simulink model "plant_block_Conrad"  (R2019b)
settings: Solver=ode1  StartTime=0.0  StopTime=700  RelTol=1e-3  EnableMultiTasking=on
undefined symbols (not defined in the file or in its folder): K4
libraries: simulink x8
settings Model: SimulationMode=external  Creator=Dro  LastModifiedBy=s4479115
settings DataIOCC: LimitDataPoints=on  SaveFormat=Array  ReturnWorkspaceOutputs=off  SignalLoggingName=sigsOut
settings OptimizationCC: ExpressionDepthLimit=2147483647  InitFltsAndDblsToZero=on
settings DebuggingCC: SaveWithParameterizedLinksMsg=none  UnderspecifiedInitializationDetection=Classic  MergeDetectMultiDrivingBlocksExec=none  SignalResolutionControl=TryResolveAllWithWarning  MultiTaskDSMMsg=warning  MultiTaskCondExecSysMsg=none  FcnCallInpInsideContextMsg=warning  StateNameClashWarn=warning  SFUnexpectedBacktrackingDiag=warning  SFNoUnconditionalDefaultTransitionDiag=warning  SFExecutionAtInitializationDiag=none  ArithmeticOperatorsInVariantConditions=warning
settings HardwareCC: TargetBitPerLong=64  TargetBitPerPointer=64  TargetIntDivRoundTo=Zero  TargetEndianess=LittleEndian  TargetWordSize=64  TargetHWDeviceType=Intel->x86-64
settings ModelReferenceCC: PropagateSignalLabelsOutOfModel=off
settings SFSimCC: SimUseLocalCustomCode=off  CustomCodeUndefinedFunction=UseInterfaceOnly
settings RTWCC: Description=Simulink Desktop Real-Time  SystemTargetFile=sldrt.tlc  TemplateMakefile=sldrt.tmf  RTWUseLocalCustomCode=off  RTWCompilerOptimization=on
settings CodeAppCC: MaxIdLength=95  StateflowObjectComments=on
settings SimulinkDesktopRealTimeCC: TargetPreCompLibLocation=C:\Program Files\MATLAB\R2019b\toolbox\sldrt\lib\win64  TargetLangStandard=C89/C90 (ANSI)  ModelReferenceCompliant=off  CompOptLevelCompliant=off  SupportVariableSizeSignals=off  PreserveStateflowLocalDataDimensions=off
settings ConfigComp: CovMetricSettings=dw  CovHtmlReporting=on  CovSaveCumulativeToWorkspaceVar=on  CovSaveSingleToWorkspaceVar=on  CovExternalEMLEnable=off

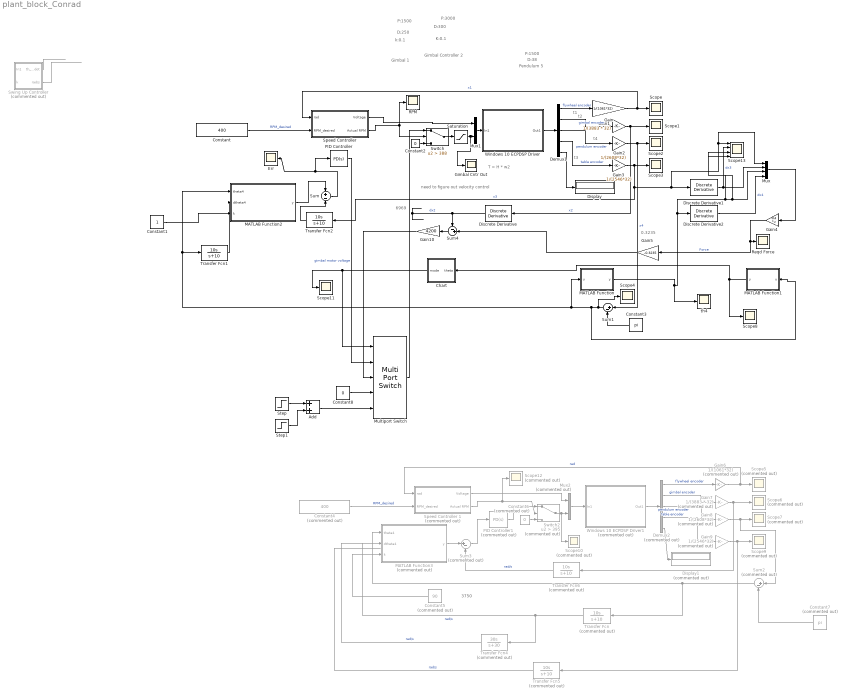
== system plant_block_Conrad ==
  note: 6969
  note: need to figure out velocity control
  note: 3750
  note: Pendulum 5
  note: D:38
  note: P:1500
  note: 0.3235
  note: t3
  note: t4
  note: t2
  note: t1
  note: T = H * w2
  note: Gimbal Controller 2
  note: K:0.1
  note: D:300
  note: P:3000
  note: Gimbal 1
  note: k:0.1
  note: D:250
  note: P:1500
  Add : Sum
  Chart : Stateflow chart  BlockKeywords=__PRM__SERIALIZED__DATA__:Stateflow Chart,Stateflow Diagram  TreatAsAtomicUnit=on
  Constant : Constant  Value=400
  Constant1 : Constant
  Constant2 : Constant  Value=0
  Constant3 : Constant  Value=pi
  Constant4 : Constant  Commented=on  Value=400
  Constant5 : Constant  Commented=on  Value=90  VectorParams1D=off
  Constant6 : Constant  Commented=on  Value=0
  Constant7 : Constant  Commented=on  Value=pi
  Constant8 : Constant  Value=0
  Demux1 : Demux  Outputs=5
  Demux2 : Demux  Commented=on  Outputs=5
  Discrete Derivative : simulink/Discrete/Discrete Derivative  gainval=1.0  ICPrevScaledInput=0.0  OutMin=[]  OutMax=[]  OutDataType=fixdt(1, 16)  OutScaling=2^-10  DoSatur=off
  Discrete Derivative1 : simulink/Discrete/Discrete Derivative  gainval=1.0  ICPrevScaledInput=0.0  OutMin=[]  OutMax=[]  OutDataType=fixdt(1, 16)  OutScaling=2^-10  DoSatur=off
  Discrete Derivative2 : simulink/Discrete/Discrete Derivative  gainval=1.0  ICPrevScaledInput=0.0  OutMin=[]  OutMax=[]  OutDataType=fixdt(1, 16)  OutScaling=2^-10  DoSatur=off
  Display : Display
  Display1 : Display  Commented=on
  Err : Scope
  Gain : Gain  Gain=1/(1061*32)
  Gain1 : Gain  Gain=1/(3883 * 32)
  Gain10 : Gain  Gain=4200
  Gain2 : Gain  Gain=1/(2608*32)
  Gain3 : Gain  Gain=1/(2546*32)
  Gain4 : Gain  Gain=-K4  Multiplication=Matrix(K*u)
  Gain5 : Gain  Gain=-0.3235
  Gain6 : Gain  Commented=on  Gain=1/(1061*32)
  Gain7 : Gain  Commented=on  Gain=1/(3883 * 32)
  Gain8 : Gain  Commented=on  Gain=1/(2608*32)
  Gain9 : Gain  Commented=on  Gain=1/(2546*32)
  Gimbal Cntr Out : Scope
  MATLAB Function : MATLAB Function  TreatAsAtomicUnit=on
  MATLAB Function1 : MATLAB Function  TreatAsAtomicUnit=on
  MATLAB Function2 : MATLAB Function  TreatAsAtomicUnit=on
  MATLAB Function3 : MATLAB Function  Commented=on  TreatAsAtomicUnit=on
  Multiport Switch : MultiPortSwitch  Inputs=4
  Mux : Mux
  Mux1 : Mux  Inputs=2
  Mux2 : Mux  Commented=on  Inputs=2
  PID Controller : simulink/Continuous/PID Controller  Controller=PD  Form=Parallel  TimeDomain=Continuous-time  SampleTime=-1  IntegratorMethod=Forward Euler  FilterMethod=Forward Euler  ControllerParametersSource=internal  P=4000  I=0  D=0  UseFilter=on  N=100  TunerSelectOption=Transfer Function Based (PID Tuner App)  InitialConditionSource=internal  InitialConditionForIntegrator=0  InitialConditionForFilter=0  DifferentiatorICPrevScaledInput=0  ExternalReset=none  TrackingMode=off  Kt=1  LimitOutput=off  UpperSaturationLimit=inf  LowerSaturationLimit=-inf  LinearizeAsGain=on  AntiWindupMode=none  Kb=1  POutMin=[]  POutMax=[]  IOutMin=[]  IOutMax=[]  DOutMin=[]  DOutMax=[]  NOutMin=[]  NOutMax=[]  SumOutMin=[]  SumOutMax=[]  SaturationOutMin=[]  SaturationOutMax=[]  PParamMin=[]  PParamMax=[]  IParamMin=[]  IParamMax=[]  DParamMin=[]  DParamMax=[]  NParamMin=[]  NParamMax=[]  KbParamMin=[]  KbParamMax=[]  KtParamMin=[]  KtParamMax=[]  KbOutMin=[]  KbOutMax=[]  KtOutMin=[]  KtOutMax=[]  IntegratorOutMin=[]  IntegratorOutMax=[]  FilterOutMin=[]  FilterOutMax=[]  SumI1OutMin=[]  SumI1OutMax=[]  SumI2OutMin=[]  SumI2OutMax=[]  SumI3OutMin=[]  SumI3OutMax=[]  SumI4OutMin=[]  SumI4OutMax=[]  SumDOutMin=[]  SumDOutMax=[]  DifferentiatorOutMin=[]  DifferentiatorOutMax=[]  FilterDiffOutCoefMin=[]  FilterDiffOutCoefMax=[]  ReciprocalOutMin=[]  ReciprocalOutMax=[]  SumDenOutMin=[]  SumDenOutMax=[]  SumNumOutMin=[]  SumNumOutMax=[]  DivideOutMin=[]  DivideOutMax=[]  IntegratorContinuousStateAttributes=''  IntegratorStateMustResolveToSignalObject=off  IntegratorRTWStateStorageClass=Auto  FilterContinuousStateAttributes=''  FilterStateMustResolveToSignalObject=off  FilterRTWStateStorageClass=Auto  ParallelPVariant=InternalParameters  IdealPVariant=Disabled  IVariant=Disabled  DVariant=InternalParameters  IntegratorVariant=Disabled  SatVariant=Disabled  AWVariant=Disabled  PCopyVariant=Disabled  TRVariant=Disabled  FdbkBlocksVariant=Forward  IdealPFdbkVariant=Disabled  SatFdbkVariant=Disabled  DerivativeFilterVariant=ContFilter  NVariant=InternalParameters  NCopyVariant=Disabled  FilterICVariant=InternalICsFilter  IntegratorICVariant=Disabled  ExternalResetVariant=Disabled  TRSumVariant=Passthrough  SumFdbkVariant=Disabled  SumVariant=Sum_PD
  PID Controller1 : simulink/Continuous/PID Controller  Commented=on  Controller=PD  Form=Parallel  TimeDomain=Continuous-time  SampleTime=-1  IntegratorMethod=Forward Euler  FilterMethod=Forward Euler  ControllerParametersSource=internal  P=40  I=1  D=0.05  UseFilter=on  N=100  TunerSelectOption=Transfer Function Based (PID Tuner App)  InitialConditionSource=internal  InitialConditionForIntegrator=0  InitialConditionForFilter=0  DifferentiatorICPrevScaledInput=0  ExternalReset=none  TrackingMode=off  Kt=1  LimitOutput=off  UpperSaturationLimit=inf  LowerSaturationLimit=-inf  LinearizeAsGain=on  AntiWindupMode=none  Kb=1  POutMin=[]  POutMax=[]  IOutMin=[]  IOutMax=[]  DOutMin=[]  DOutMax=[]  NOutMin=[]  NOutMax=[]  SumOutMin=[]  SumOutMax=[]  SaturationOutMin=[]  SaturationOutMax=[]  PParamMin=[]  PParamMax=[]  IParamMin=[]  IParamMax=[]  DParamMin=[]  DParamMax=[]  NParamMin=[]  NParamMax=[]  KbParamMin=[]  KbParamMax=[]  KtParamMin=[]  KtParamMax=[]  KbOutMin=[]  KbOutMax=[]  KtOutMin=[]  KtOutMax=[]  IntegratorOutMin=[]  IntegratorOutMax=[]  FilterOutMin=[]  FilterOutMax=[]  SumI1OutMin=[]  SumI1OutMax=[]  SumI2OutMin=[]  SumI2OutMax=[]  SumI3OutMin=[]  SumI3OutMax=[]  SumI4OutMin=[]  SumI4OutMax=[]  SumDOutMin=[]  SumDOutMax=[]  DifferentiatorOutMin=[]  DifferentiatorOutMax=[]  FilterDiffOutCoefMin=[]  FilterDiffOutCoefMax=[]  ReciprocalOutMin=[]  ReciprocalOutMax=[]  SumDenOutMin=[]  SumDenOutMax=[]  SumNumOutMin=[]  SumNumOutMax=[]  DivideOutMin=[]  DivideOutMax=[]  IntegratorContinuousStateAttributes=''  IntegratorStateMustResolveToSignalObject=off  IntegratorRTWStateStorageClass=Auto  FilterContinuousStateAttributes=''  FilterStateMustResolveToSignalObject=off  FilterRTWStateStorageClass=Auto  ParallelPVariant=InternalParameters  IdealPVariant=Disabled  IVariant=Disabled  DVariant=InternalParameters  IntegratorVariant=Disabled  SatVariant=Disabled  AWVariant=Disabled  PCopyVariant=Disabled  TRVariant=Disabled  FdbkBlocksVariant=Forward  IdealPFdbkVariant=Disabled  SatFdbkVariant=Disabled  DerivativeFilterVariant=ContFilter  NVariant=InternalParameters  NCopyVariant=Disabled  FilterICVariant=InternalICsFilter  IntegratorICVariant=Disabled  ExternalResetVariant=Disabled  TRSumVariant=Passthrough  SumFdbkVariant=Disabled  SumVariant=Sum_PD
  "RPM " : Scope
  Reqd Force : Scope
  Saturation : Saturate  UpperLimit=16000  LowerLimit=-16000
  Scope{,1..4,8,11} (7 alike) : Scope
  Scope{5..7,9..10,12} (6 alike) : Scope  Commented=on
  Scope13 : Scope  NumInputPorts=4
  "Speed Controller " : Subsystem
  Speed Controller 1 : Subsystem  Commented=on
  Step : Step  Time=30  After=3000  SampleTime=0
  Step1 : Step  Time=30.2  Before=3000  After=-3000  SampleTime=0
  Sum : Sum  Inputs=+-
  Sum1 : Sum  Inputs=|+-
  Sum2 : Sum  Commented=on  Inputs=|+-
  Sum3 : Sum  Commented=on  Inputs=|+-
  Sum4 : Sum  Inputs=-+|
  "Swing Up Controller " : Subsystem  Commented=on
  Switch : Switch  Criteria=u2 > Threshold  Threshold=388
  Switch2 : Switch  Commented=on  Criteria=u2 > Threshold  Threshold=395
  Transfer Fcn : TransferFcn  Commented=on  Numerator=[10 0 ]  Denominator=[1 10]
  Transfer Fcn1 : TransferFcn  Numerator=[10 0]  Denominator=[1 10]
  Transfer Fcn2 : TransferFcn  Numerator=[10 0]  Denominator=[1 10]
  Transfer Fcn4 : TransferFcn  Commented=on  Numerator=[30 0 ]  Denominator=[1 30]
  Transfer Fcn5 : TransferFcn  Commented=on  Numerator=[10 0 ]  Denominator=[1 10]
  Transfer Fcn6 : TransferFcn  Commented=on  Numerator=[10 0 ]  Denominator=[1 10]
  Windows 10 ECPDSP Driver : Subsystem  mask{BaseAddr='0x3F00', STime=0.008, TimeOutPer=500, HWAccess=on}
      mask prompts: BaseAddr "Base I/O Address"; STime "Sample Time (Sec)"; TimeOutPer "Timeout Period (500 ~ 2000)"; HWAccess "Hardware Access"
      mask Display: color('black');disp('ECPDSP Driver\n upto\n 4 Encs(ADC Channels)\n and 2 Dacs')
  Windows 10 ECPDSP Driver1 : Subsystem  Commented=on  mask{BaseAddr='0x3F00', STime=0.008, TimeOutPer=500, HWAccess=on}
      mask prompts: BaseAddr "Base I/O Address"; STime "Sample Time (Sec)"; TimeOutPer "Timeout Period (500 ~ 2000)"; HWAccess "Hardware Access"
      mask Display: color('black');disp('ECPDSP Driver\n upto\n 4 Encs(ADC Channels)\n and 2 Dacs')
  th4 : Scope
  wires:
  Mux1/1 -> Windows 10 ECPDSP Driver/1(In1)
  Demux1/1 -> Gain/1  "flywheel encoder"
  Demux1/2 -> Gain1/1  "gimbal encoder"
  Demux1/3 -> Gain2/1  "pendulum encoder"
  Demux1/4 -> Gain3/1  "table encoder"
  Gain4/1 -> Gain5/1, Reqd Force/1  "Force"
  Windows 10 ECPDSP Driver/1(Out1) -> Demux1/1
  Demux1/5 -> Display/1
  Gain/1 -> "Speed Controller "/1(rad), Scope/1  "x1"
  Gain1/1 -> Discrete Derivative/1, Scope1/1  "x2"
  Gain3/1 -> Transfer Fcn2/1, Discrete Derivative1/1, Scope13/1, Mux/1, Scope3/1  "x3"
  Constant/1 -> "Speed Controller "/2(RPM_desired)  "RPM_desired"
  "Speed Controller "/1(Voltage) -> Mux1/1
  "Speed Controller "/2("Actual RPM ") -> "RPM "/1, Switch/2
  Constant2/1 -> Switch/3
  Constant3/1 -> Sum1/2
  Gain2/1 -> Sum1/1, Scope2/1  "x4"
  Discrete Derivative2/1 -> Mux/4  "dx4"
  Discrete Derivative1/1 -> Scope13/2, Mux/2  "dx3"
  Mux/1 -> Gain4/1
  MATLAB Function1/1(y) -> Chart/1(theta), Scope8/1
  PID Controller/1 -> Multiport Switch/2  "gimbal motor voltage"
  Discrete Derivative/1 -> Sum4/1  "dx2"
  Gain5/1 -> Sum4/2
  "Swing Up Controller "/1(th_2_dot) -> ?
  Constant1/1 -> MATLAB Function2/3(k)
  "Swing Up Controller "/2(rad/s) -> ?
  Chart/1(mode) -> Multiport Switch/1, Scope11/1
  Sum/1 -> Err/1, PID Controller/1
  Sum1/1 -> Scope4/1, MATLAB Function2/1(theta4), Transfer Fcn1/1, MATLAB Function/1(u), MATLAB Function1/1(u)
  MATLAB Function/1(y) -> th4/1, Discrete Derivative2/1, Scope13/3, Scope13/4, Mux/3
  Speed Controller 1/1(Voltage) -> Mux2/1
  Transfer Fcn5/1 -> ?  "rad/s"
  Gain9/1 -> Transfer Fcn5/1, Scope9/1
  Transfer Fcn4/1 -> ?  "rad/s"
  Transfer Fcn/1 -> MATLAB Function3/2(dtheta4), Transfer Fcn4/1  "rad/s"
  Mux2/1 -> Windows 10 ECPDSP Driver1/1(In1)
  Demux2/3 -> Gain8/1  "pendulum encoder"
  Windows 10 ECPDSP Driver1/1(Out1) -> Demux2/1
  Constant4/1 -> Speed Controller 1/2(RPM_desired)  "RPM_desired"
  Gain6/1 -> Speed Controller 1/1(rad), Scope5/1  "rad"
  Sum2/1 -> MATLAB Function3/1(theta4), Transfer Fcn/1
  Switch2/1 -> Scope10/1, Mux2/2
  Speed Controller 1/2("Actual RPM ") -> Scope12/1, Switch2/2
  Demux2/2 -> Gain7/1  "gimbal encoder"
  Demux2/4 -> Gain9/1  "table encoder"
  Demux2/5 -> Display1/1
  Gain7/1 -> Transfer Fcn6/1, Scope6/1
  Constant6/1 -> Switch2/3
  Constant5/1 -> MATLAB Function3/3(k)
  Gain8/1 -> Scope7/1, Sum2/1
  Constant7/1 -> Sum2/2
  Demux2/1 -> Gain6/1  "flywheel encoder"
  MATLAB Function3/1(y) -> Sum3/1
  PID Controller1/1 -> Switch2/1
  Sum3/1 -> PID Controller1/1
  Transfer Fcn6/1 -> Sum3/2  "rad/s"
  Gain10/1 -> Multiport Switch/3
  Multiport Switch/1 -> Switch/1
  Switch/1 -> Saturation/1
  Saturation/1 -> Gimbal Cntr Out/1, Mux1/2
  Sum4/1 -> Gain10/1
  MATLAB Function2/1(y) -> Sum/1
  Transfer Fcn1/1 -> MATLAB Function2/2(dtheta4)
  Transfer Fcn2/1 -> Sum/2
  Constant8/1 -> Multiport Switch/4
  Add/1 -> Multiport Switch/5
  Step/1 -> Add/1
  Step1/1 -> Add/2

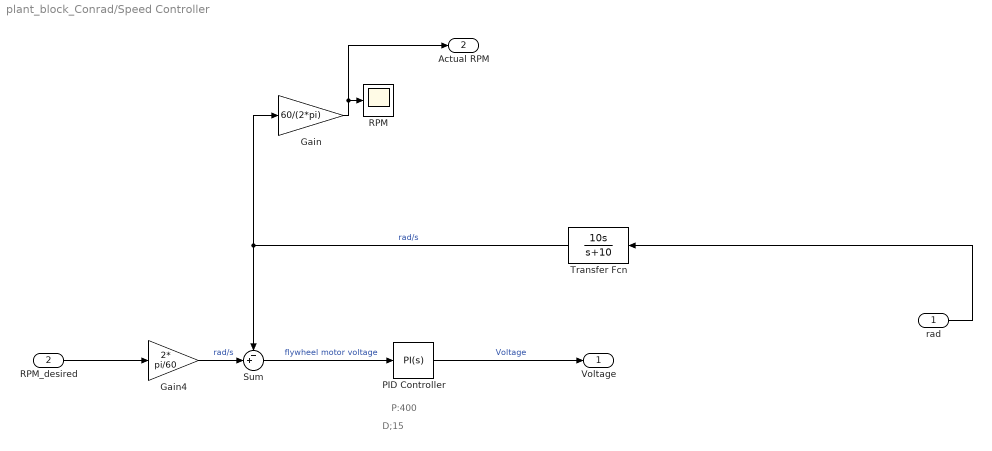
== system plant_block_Conrad/Speed Controller  ==
  note: D;15
  note: P:400
  rad : Inport
  RPM_desired : Inport  Port=2
  Gain : Gain  Gain=60/(2*pi)
  Gain4 : Gain  Gain=2* pi/60
  PID Controller : simulink/Continuous/PID Controller  Controller=PI  Form=Parallel  TimeDomain=Continuous-time  SampleTime=-1  IntegratorMethod=Forward Euler  FilterMethod=Forward Euler  ControllerParametersSource=internal  P=390  I=15  D=0  UseFilter=on  N=100  TunerSelectOption=Transfer Function Based (PID Tuner App)  InitialConditionSource=internal  InitialConditionForIntegrator=0  InitialConditionForFilter=0  DifferentiatorICPrevScaledInput=0  ExternalReset=none  TrackingMode=off  Kt=1  LimitOutput=off  UpperSaturationLimit=inf  LowerSaturationLimit=-inf  LinearizeAsGain=on  AntiWindupMode=none  Kb=1  POutMin=[]  POutMax=[]  IOutMin=[]  IOutMax=[]  DOutMin=[]  DOutMax=[]  NOutMin=[]  NOutMax=[]  SumOutMin=[]  SumOutMax=[]  SaturationOutMin=[]  SaturationOutMax=[]  PParamMin=[]  PParamMax=[]  IParamMin=[]  IParamMax=[]  DParamMin=[]  DParamMax=[]  NParamMin=[]  NParamMax=[]  KbParamMin=[]  KbParamMax=[]  KtParamMin=[]  KtParamMax=[]  KbOutMin=[]  KbOutMax=[]  KtOutMin=[]  KtOutMax=[]  IntegratorOutMin=[]  IntegratorOutMax=[]  FilterOutMin=[]  FilterOutMax=[]  SumI1OutMin=[]  SumI1OutMax=[]  SumI2OutMin=[]  SumI2OutMax=[]  SumI3OutMin=[]  SumI3OutMax=[]  SumI4OutMin=[]  SumI4OutMax=[]  SumDOutMin=[]  SumDOutMax=[]  DifferentiatorOutMin=[]  DifferentiatorOutMax=[]  FilterDiffOutCoefMin=[]  FilterDiffOutCoefMax=[]  ReciprocalOutMin=[]  ReciprocalOutMax=[]  SumDenOutMin=[]  SumDenOutMax=[]  SumNumOutMin=[]  SumNumOutMax=[]  DivideOutMin=[]  DivideOutMax=[]  IntegratorContinuousStateAttributes=''  IntegratorStateMustResolveToSignalObject=off  IntegratorRTWStateStorageClass=Auto  FilterContinuousStateAttributes=''  FilterStateMustResolveToSignalObject=off  FilterRTWStateStorageClass=Auto  ParallelPVariant=InternalParameters  IdealPVariant=Disabled  IVariant=InternalParameters  DVariant=Disabled  IntegratorVariant=Continuous  SatVariant=Disabled  AWVariant=Passthrough  PCopyVariant=Disabled  TRVariant=Disabled  FdbkBlocksVariant=Forward  IdealPFdbkVariant=Disabled  SatFdbkVariant=Disabled  DerivativeFilterVariant=Disabled  NVariant=Disabled  NCopyVariant=Disabled_SignalSpec  FilterICVariant=Disabled  IntegratorICVariant=InternalICs  ExternalResetVariant=Disabled  TRSumVariant=Passthrough  SumFdbkVariant=Disabled  SumVariant=Sum_PI
  RPM : Scope
  Sum : Sum  Inputs=-+|
  Transfer Fcn : TransferFcn  Numerator=[10 0 ]  Denominator=[1 10]
  Voltage : Outport
  "Actual RPM " : Outport  Port=2
  wires:
  Gain4/1 -> Sum/2  "rad/s"
  Transfer Fcn/1 -> Gain/1, Sum/1  "rad/s"
  Sum/1 -> PID Controller/1  "flywheel motor voltage"
  PID Controller/1 -> Voltage/1  "Voltage"
  RPM_desired/1 -> Gain4/1
  rad/1 -> Transfer Fcn/1
  Gain/1 -> "Actual RPM "/1, RPM/1

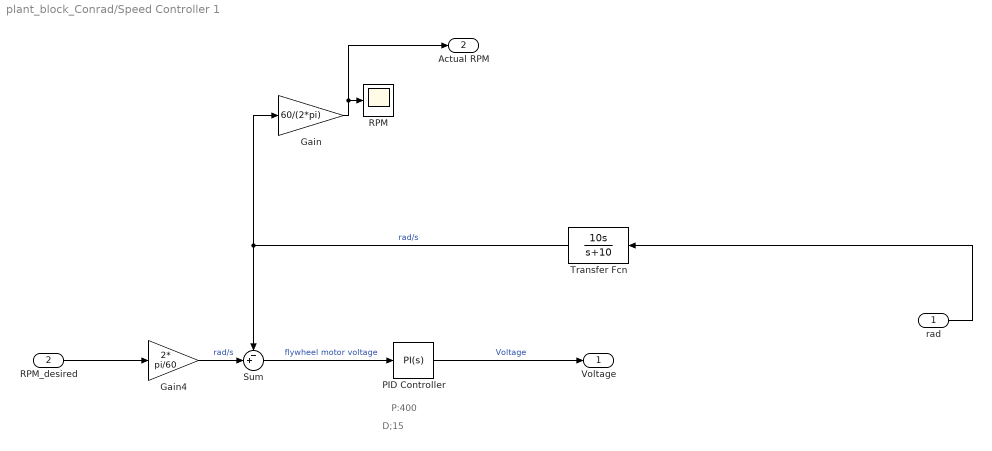
== system plant_block_Conrad/Speed Controller 1 ==
  note: D;15
  note: P:400
  rad : Inport
  RPM_desired : Inport  Port=2
  Gain : Gain  Gain=60/(2*pi)
  Gain4 : Gain  Gain=2* pi/60
  PID Controller : simulink/Continuous/PID Controller  Controller=PI  Form=Parallel  TimeDomain=Continuous-time  SampleTime=-1  IntegratorMethod=Forward Euler  FilterMethod=Forward Euler  ControllerParametersSource=internal  P=600  I=50  D=0  UseFilter=on  N=100  TunerSelectOption=Transfer Function Based (PID Tuner App)  InitialConditionSource=internal  InitialConditionForIntegrator=0  InitialConditionForFilter=0  DifferentiatorICPrevScaledInput=0  ExternalReset=none  TrackingMode=off  Kt=1  LimitOutput=off  UpperSaturationLimit=inf  LowerSaturationLimit=-inf  LinearizeAsGain=on  AntiWindupMode=none  Kb=1  POutMin=[]  POutMax=[]  IOutMin=[]  IOutMax=[]  DOutMin=[]  DOutMax=[]  NOutMin=[]  NOutMax=[]  SumOutMin=[]  SumOutMax=[]  SaturationOutMin=[]  SaturationOutMax=[]  PParamMin=[]  PParamMax=[]  IParamMin=[]  IParamMax=[]  DParamMin=[]  DParamMax=[]  NParamMin=[]  NParamMax=[]  KbParamMin=[]  KbParamMax=[]  KtParamMin=[]  KtParamMax=[]  KbOutMin=[]  KbOutMax=[]  KtOutMin=[]  KtOutMax=[]  IntegratorOutMin=[]  IntegratorOutMax=[]  FilterOutMin=[]  FilterOutMax=[]  SumI1OutMin=[]  SumI1OutMax=[]  SumI2OutMin=[]  SumI2OutMax=[]  SumI3OutMin=[]  SumI3OutMax=[]  SumI4OutMin=[]  SumI4OutMax=[]  SumDOutMin=[]  SumDOutMax=[]  DifferentiatorOutMin=[]  DifferentiatorOutMax=[]  FilterDiffOutCoefMin=[]  FilterDiffOutCoefMax=[]  ReciprocalOutMin=[]  ReciprocalOutMax=[]  SumDenOutMin=[]  SumDenOutMax=[]  SumNumOutMin=[]  SumNumOutMax=[]  DivideOutMin=[]  DivideOutMax=[]  IntegratorContinuousStateAttributes=''  IntegratorStateMustResolveToSignalObject=off  IntegratorRTWStateStorageClass=Auto  FilterContinuousStateAttributes=''  FilterStateMustResolveToSignalObject=off  FilterRTWStateStorageClass=Auto  ParallelPVariant=InternalParameters  IdealPVariant=Disabled  IVariant=InternalParameters  DVariant=Disabled  IntegratorVariant=Continuous  SatVariant=Disabled  AWVariant=Passthrough  PCopyVariant=Disabled  TRVariant=Disabled  FdbkBlocksVariant=Forward  IdealPFdbkVariant=Disabled  SatFdbkVariant=Disabled  DerivativeFilterVariant=Disabled  NVariant=Disabled  NCopyVariant=Disabled_SignalSpec  FilterICVariant=Disabled  IntegratorICVariant=InternalICs  ExternalResetVariant=Disabled  TRSumVariant=Passthrough  SumFdbkVariant=Disabled  SumVariant=Sum_PI
  RPM : Scope
  Sum : Sum  Inputs=-+|
  Transfer Fcn : TransferFcn  Numerator=[10 0 ]  Denominator=[1 10]
  Voltage : Outport
  "Actual RPM " : Outport  Port=2
  wires:
  Gain4/1 -> Sum/2  "rad/s"
  Transfer Fcn/1 -> Gain/1, Sum/1  "rad/s"
  Sum/1 -> PID Controller/1  "flywheel motor voltage"
  PID Controller/1 -> Voltage/1  "Voltage"
  RPM_desired/1 -> Gain4/1
  rad/1 -> Transfer Fcn/1
  Gain/1 -> "Actual RPM "/1, RPM/1

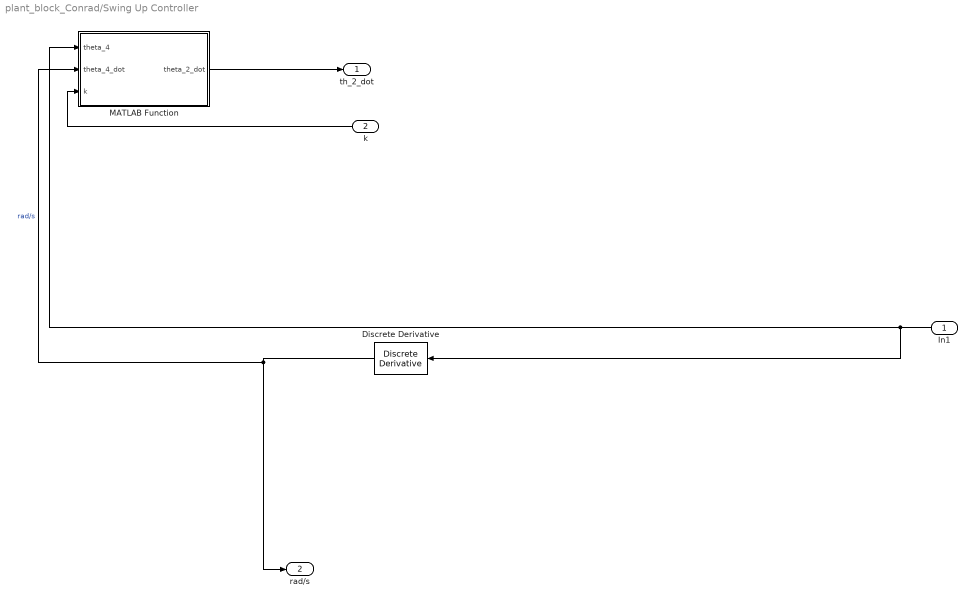
== system plant_block_Conrad/Swing Up Controller  ==
  In1 : Inport
  k : Inport  Port=2
  Discrete Derivative : simulink/Discrete/Discrete Derivative  gainval=1.0  ICPrevScaledInput=0.0  OutMin=[]  OutMax=[]  OutDataType=fixdt(1, 16)  OutScaling=2^-10  DoSatur=off
  MATLAB Function : MATLAB Function  TreatAsAtomicUnit=on
  th_2_dot : Outport
  rad/s : Outport  Port=2
  wires:
  MATLAB Function/1(theta_2_dot) -> th_2_dot/1
  k/1 -> MATLAB Function/3(k)
  Discrete Derivative/1 -> rad/s/1, MATLAB Function/2(theta_4_dot)  "rad/s"
  In1/1 -> Discrete Derivative/1, MATLAB Function/1(theta_4)

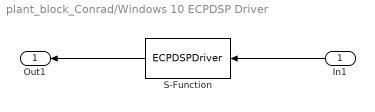
== system plant_block_Conrad/Windows 10 ECPDSP Driver ==
  In1 : Inport
  S-Function : S-Function  FunctionName=ECPDSPDriver  Parameters=BaseAddr,STime,TimeOutPer,HWAccess  SFunctionDeploymentMode=off  EnableBusSupport=off
  Out1 : Outport
  wires:
  In1/1 -> S-Function/1
  S-Function/1 -> Out1/1

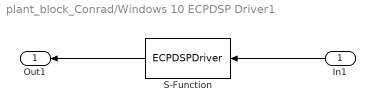
== system plant_block_Conrad/Windows 10 ECPDSP Driver1 ==
  In1 : Inport
  S-Function : S-Function  FunctionName=ECPDSPDriver  Parameters=BaseAddr,STime,TimeOutPer,HWAccess  SFunctionDeploymentMode=off  EnableBusSupport=off
  Out1 : Outport
  wires:
  In1/1 -> S-Function/1
  S-Function/1 -> Out1/1

== matlab function plant_block_Conrad/MATLAB Function1 ==
  data: u input; y output
function y = fcn(u)

y = min( abs(mod(u, 2 * pi)) , abs(mod(u, 2* pi) - 2 * pi));

== matlab function plant_block_Conrad/Swing Up Controller /MATLAB Function ==
  data: theta_4 input; theta_2_dot output; theta_4_dot input; k input
function theta_2_dot = fcn(theta_4, theta_4_dot, k)

theta_2_dot = -(36353776222982492160*k*theta_4_dot*cos(theta_4)*((3314449799178915*theta_4_dot^2)/576460752303423488 + (7532743254738029*cos(theta_4))/18014398509481984 - 7532743254738029/18014398509481984))/(299580375726665093*pi);
% theta_2_dot = -0.5722*k*theta_4_dot*cos(theta_4)*(0.0057*theta_4_dot^2 + 0.4182*cos(theta_4) - 0.4182);
end

== stateflow chart plant_block_Conrad/Chart ==
  state Spool1
    mode=3
  state Kick
    mode=4
  state Swing_up
    mode=1
  state Capture
    mode=2
  state Reset
    mode=3
  (default) -> Spool1
  Spool1 -> Kick : after(30000, msec)
  Swing_up -> Capture : [abs(theta)<0.08]
  Capture -> Reset : [abs(theta)>0.15]
  Kick -> Swing_up : after(500, msec)
  Reset -> Swing_up : after(3000, msec)
  data: mode output; theta input

== matlab function plant_block_Conrad/MATLAB Function ==
  data: u input; y output
function y = mabs(u)
% th = abs(u);
th1 = mod(u, 2 * pi);
th2 = 2*pi - th1;
arr = [th1, -th2];
[minMag, index] = min(abs(arr(:)));
y = minMag * sign(arr(index));
end

== matlab function plant_block_Conrad/MATLAB Function2 ==
  data: theta4 input; y output; dtheta4 input; k input
function y = fcn(theta4, dtheta4,k)
m = 0.1580;
lcg = 0.2698;
rh = 0.37;
J1 = 0.1314;
Jz_bar = 0.0131;
g = 9.81;
c = 0.002;
Eo = 0;
Id = 0.0148;
dtheta1 = 400 * (2*pi/60);

E = 0.5*m*lcg^2*dtheta4^2 + m*g*lcg*(cos(theta4) - 1);

% might need to negate k...simulation says so...???
y = -k*(E - Eo)*dtheta4*cos(theta4);

% dtheta2 = (rh/(Id*dtheta1))*...
%     ((J1+m*rh^2)*ddtheta3 + m*lcg*rh*cos(theta4)*ddtheta4 - ...
%     m*lcg*rh*sin(theta4)*dtheta4^2 + c*dtheta3);
end

== matlab function plant_block_Conrad/MATLAB Function3 ==
  data: theta4 input; y output; dtheta4 input; k input
function y = fcn(theta4, dtheta4,k)
m = 0.1580;
lcg = 0.2698;
rh = 0.37;
J1 = 0.1314;
Jz_bar = 0.0131;
g = 9.81;
c = 0.002;
Eo = 0;
Id = 0.0148;
dtheta1 = 400 * (2*pi/60);

E = 0.5*m*lcg^2*dtheta4^2 + m*g*lcg*(cos(theta4) - 1);

% might need to negate k...simulation says so...???
y = -k*(E - Eo)*dtheta4*cos(theta4);

% dtheta2 = (rh/(Id*dtheta1))*...
%     ((J1+m*rh^2)*ddtheta3 + m*lcg*rh*cos(theta4)*ddtheta4 - ...
%     m*lcg*rh*sin(theta4)*dtheta4^2 + c*dtheta3);
end
